simulink subsystem "ttc_on_road"  (R2022b)
settings: Solver=VariableStepAuto  StartTime=0.0  StopTime=10.0  RelTol=1e-3
settings Model: Creator=USER  LastModifiedBy=USER

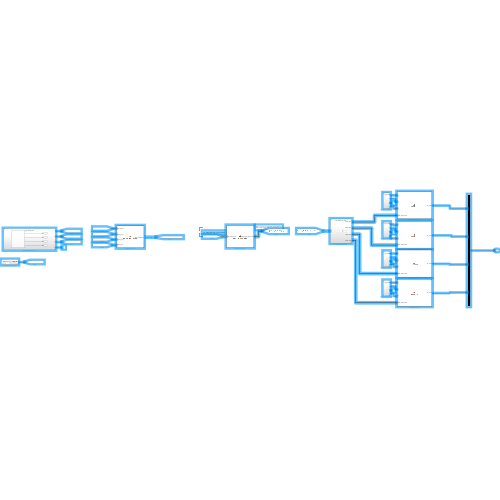
[thumbnail: Simulink's stored preview of the top-level diagram]
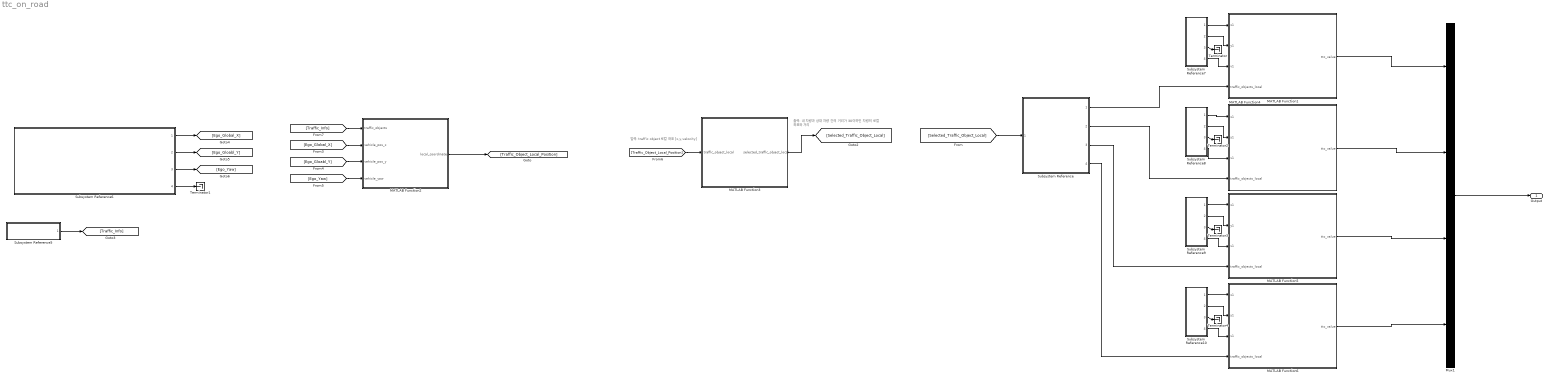
== system ttc_on_road ==
  note: 출력: 내 차량과 상대 차량 간의 거리가 30이하인 차령의 로컬 좌표와 거리
  note: 입력: traffic object 로컬 좌표 [x,y,velocity]
  MATLAB Function1 : MATLAB Function  TreatAsAtomicUnit=on
  MATLAB Function2 : MATLAB Function  TreatAsAtomicUnit=on
  MATLAB Function3 : MATLAB Function  TreatAsAtomicUnit=on
  MATLAB Function4 : MATLAB Function  TreatAsAtomicUnit=on
  MATLAB Function5 : MATLAB Function  TreatAsAtomicUnit=on
  MATLAB Function6 : MATLAB Function  TreatAsAtomicUnit=on
  Mux1 : Mux
  Subsystem Reference : Subsystem  ReferencedSubsystem=Get_Traffic_by_Line
  Subsystem Reference{6..10} (5 alike) : Subsystem  ReferencedSubsystem=ego_vehicle_info
  Subsystem Reference5 : Subsystem  ReferencedSubsystem=traffic_object_on_road_info
  Terminator{,1..4} (5 alike) : Terminator
  Output : Outport
  wires:
  Subsystem Reference7/4 -> MATLAB Function1/3(v1)
  Subsystem Reference7/1 -> MATLAB Function1/1(x1)
  MATLAB Function3/1(selected_traffic_object_local) -> [Selected_Traffic_Object_Local]
  MATLAB Function2/1(local_coordinates) -> [Traffic_Object_Local_Position]
  [Ego_Gloabl_Y] -> MATLAB Function2/3(vehicle_pos_y)
  Subsystem Reference6/3 -> [Ego_Yaw]
  [Traffic_Object_Local_Position] -> MATLAB Function3/1(traffic_object_local)
  Subsystem Reference10/1 -> MATLAB Function6/1(x1)
  MATLAB Function6/1(ttc_value) -> Mux1/4
  Subsystem Reference/1 -> MATLAB Function1/4(traffic_objects_local)
  Subsystem Reference/4 -> MATLAB Function6/4(traffic_objects_local)
  Subsystem Reference/2 -> MATLAB Function4/4(traffic_objects_local)
  Subsystem Reference8/2 -> MATLAB Function4/2(y1)
  Subsystem Reference7/3 -> Terminator/1
  Subsystem Reference8/4 -> MATLAB Function4/3(v1)
  Subsystem Reference9/3 -> Terminator3/1
  Subsystem Reference5/1 -> [Traffic_Info]
  Subsystem Reference10/3 -> Terminator4/1
  MATLAB Function4/1(ttc_value) -> Mux1/2
  Subsystem Reference8/1 -> MATLAB Function4/1(x1)
  MATLAB Function1/1(ttc_value) -> Mux1/1
  Subsystem Reference7/2 -> MATLAB Function1/2(y1)
  Subsystem Reference9/1 -> MATLAB Function5/1(x1)
  Subsystem Reference9/4 -> MATLAB Function5/3(v1)
  Subsystem Reference6/4 -> Terminator1/1
  Subsystem Reference/3 -> MATLAB Function5/4(traffic_objects_local)
  Mux1/1 -> Output/1
  Subsystem Reference6/2 -> [Ego_Gloabl_Y]
  Subsystem Reference9/2 -> MATLAB Function5/2(y1)
  [Ego_Yaw] -> MATLAB Function2/4(vehicle_yaw)
  Subsystem Reference8/3 -> Terminator2/1
  Subsystem Reference10/2 -> MATLAB Function6/2(y1)
  [Ego_Global_X] -> MATLAB Function2/2(vehicle_pos_x)
  MATLAB Function5/1(ttc_value) -> Mux1/3
  [Traffic_Info] -> MATLAB Function2/1(traffic_objects)
  Subsystem Reference6/1 -> [Ego_Global_X]
  Subsystem Reference10/4 -> MATLAB Function6/3(v1)
  [Selected_Traffic_Object_Local] -> Subsystem Reference/1

== matlab function ttc_on_road/MATLAB Function2 ==
  settings: updateMethod=DISCRETE  sampleTime=0.05
  data: local_coordinates output size=[30, 3]; traffic_objects input; vehicle_pos_x input; vehicle_pos_y input; vehicle_yaw input
function local_coordinates = global_to_local_position(traffic_objects, vehicle_pos_x, vehicle_pos_y, vehicle_yaw)
    % 차량 위치를 기준으로 변환 (평행 이동)
    delta_x = traffic_objects(:,1) - vehicle_pos_x;
    delta_y = traffic_objects(:,2) - vehicle_pos_y;
    
    % 차량의 요(방향)에 따른 회전 변환
    x_l = cos(vehicle_yaw) * delta_x + sin(vehicle_yaw) * delta_y;
    y_l = -sin(vehicle_yaw) * delta_x + cos(vehicle_yaw) * delta_y;
    
    coder.varsize('local_coordinates', [30, 3]);
    local_coordinates = zeros(size(traffic_objects,1),3); % 지역 좌표를 저장할 배열

    for i = 1:size(traffic_objects,1)
        velocity =  sqrt(traffic_objects(i,3)^2 + traffic_objects(i,4)^2);
        local_coordinates(i,:) = [x_l(i), y_l(i),velocity];
    end
end
% 
% function localVelocity = globalToLocalVelocity(v_x, v_y, theta)
%     % 전역 좌표계의 속도 벡터를 로컬 좌표계로 변환
%     %   v_x, v_y - 전역 좌표계에서의 속도 벡터 (x, y 속도)
%     %   theta - 차량의 진행 방향 (yaw angle in radians)
% 
%     v_x_l = cos(theta) * v_x + sin(theta) * v_y;
%     v_y_l = -sin(theta) * v_x + cos(theta) * v_y;
% 
%     % 회전 변환을 적용하여 로컬 속도를 계산
%     localVelocity =  sqrt(v_x_l^2 + v_y_l^2);
% end

== matlab function ttc_on_road/MATLAB Function3 ==
  settings: updateMethod=DISCRETE  sampleTime=0.05
  data: selected_traffic_object_local output size=[30, 4]; traffic_object_local input
function selected_traffic_object_local = select_near_traffic_object (traffic_object_local)
    % 차량 수
    numVehicles = size(traffic_object_local, 1);
    
    % 내 차와의 거리가 30 이하인 local cordinate를 저장할 배열
    coder.varsize('selected_traffic_object_local', [30, 4]);
    selected_traffic_object_local = zeros(0,4); 

    % 각 차량과의 거리 계산 및 거리가 30이하인 경우 출력으로 보냄
    for i = 1:numVehicles
        x = traffic_object_local(i,1);
        y = traffic_object_local(i,2);
        distance = sqrt(x^2 + y^2);

        if distance <= 30
            selected_traffic_object_local = [selected_traffic_object_local;traffic_object_local(i,:) distance];

        end
    end
end

== matlab function ttc_on_road/MATLAB Function4 ==
  settings: updateMethod=DISCRETE  sampleTime=0.05
  data: ttc_value output; x1 input; y1 input; v1 input; traffic_objects_local input
function ttc_value = calculateTTC(x1, y1, v1, traffic_objects_local)
    % 여러 상대 차량과의 Time to Collision 계산 함수
    % 입력:
    %   x1, y1 - 내 차량의 좌표
    %   v1 - 내 차량의 속도 (크기)
    %   traffic_objects_local - Nx3 행렬로, 각 행은 상대 차량의 (x, y,velocity) 좌표
    %   distance - Nx1 벡터로 내 차량과 다른 차량 사이의 거리
    % 출력:
    %   ttc_values - 각 상대 차량과의 Time to Collision 값

    % 차량 수
    numVehicles = size(traffic_objects_local, 1);

    if numVehicles > 0
        % 거리 및 TTC 저장을 위한 배열 초기화
        ttc_values = zeros(numVehicles, 1);
        
        % 각 차량과의 거리 및 상대 속도 계산
        for i = 1:numVehicles
    
            % 상대 속도 계산 (내 차량 속도와 상대 차량 속도의 차이)
            v2 = traffic_objects_local(i,3);
            relative_velocity = v2 - v1;

            % Time to Collision 계산
            if relative_velocity > 0
                ttc_values(i) = traffic_objects_local(i,4) / relative_velocity;
            else
                % 상대 속도가 0이거나 음수일 때 (멀어지는 경우 TTC는 무한대 처리)
                ttc_values(i) = inf;
            end
        end

        % 행렬에서 inf 값을 제외한 값들만 선택
        finiteValues = ttc_values(isfinite(ttc_values));
    
        % inf가 아닌 값들 중 최소 값 계산
        if ~isempty(finiteValues)
            ttc_value = min(finiteValues);
        else
            % 모든 값이 inf일 경우
            ttc_value = inf;
        end
    
    else
        ttc_value = inf;
    end
end

== matlab function ttc_on_road/MATLAB Function5 ==
  settings: updateMethod=DISCRETE  sampleTime=0.05
  data: ttc_value output; x1 input; y1 input; v1 input; traffic_objects_local input
function ttc_value = calculateTTC(x1, y1, v1, traffic_objects_local)
    % 여러 상대 차량과의 Time to Collision 계산 함수
    % 입력:
    %   x1, y1 - 내 차량의 좌표
    %   v1 - 내 차량의 속도 (크기)
    %   traffic_objects_local - Nx3 행렬로, 각 행은 상대 차량의 (x, y,velocity) 좌표
    %   distance - Nx1 벡터로 내 차량과 다른 차량 사이의 거리
    % 출력:
    %   ttc_values - 각 상대 차량과의 Time to Collision 값

    % 차량 수
    numVehicles = size(traffic_objects_local, 1);

    if numVehicles > 0
        % 거리 및 TTC 저장을 위한 배열 초기화
        ttc_values = zeros(numVehicles, 1);
        
        % 각 차량과의 거리 및 상대 속도 계산
        for i = 1:numVehicles
    
            % 상대 속도 계산 (내 차량 속도와 상대 차량 속도의 차이)
            v2 = traffic_objects_local(i,3);
            relative_velocity = v2 - v1;

            % Time to Collision 계산
            if relative_velocity > 0
                ttc_values(i) = traffic_objects_local(i,4) / relative_velocity;
            else
                % 상대 속도가 0이거나 음수일 때 (멀어지는 경우 TTC는 무한대 처리)
                ttc_values(i) = inf;
            end
        end

        % 행렬에서 inf 값을 제외한 값들만 선택
        finiteValues = ttc_values(isfinite(ttc_values));
    
        % inf가 아닌 값들 중 최소 값 계산
        if ~isempty(finiteValues)
            ttc_value = min(finiteValues);
        else
            % 모든 값이 inf일 경우
            ttc_value = inf;
        end
    
    else
        ttc_value = inf;
    end
end

== matlab function ttc_on_road/MATLAB Function6 ==
  settings: updateMethod=DISCRETE  sampleTime=0.05
  data: ttc_value output; x1 input; y1 input; v1 input; traffic_objects_local input
function ttc_value = calculateTTC(x1, y1, v1, traffic_objects_local)
    % 여러 상대 차량과의 Time to Collision 계산 함수
    % 입력:
    %   x1, y1 - 내 차량의 좌표
    %   v1 - 내 차량의 속도 (크기)
    %   traffic_objects_local - Nx3 행렬로, 각 행은 상대 차량의 (x, y,velocity) 좌표
    %   distance - Nx1 벡터로 내 차량과 다른 차량 사이의 거리
    % 출력:
    %   ttc_values - 각 상대 차량과의 Time to Collision 값

    % 차량 수
    numVehicles = size(traffic_objects_local, 1);

    if numVehicles > 0
        % 거리 및 TTC 저장을 위한 배열 초기화
        ttc_values = zeros(numVehicles, 1);
        
        % 각 차량과의 거리 및 상대 속도 계산
        for i = 1:numVehicles
    
            % 상대 속도 계산 (내 차량 속도와 상대 차량 속도의 차이)
            v2 = traffic_objects_local(i,3);
            relative_velocity = v2 - v1;

            % Time to Collision 계산
            if relative_velocity > 0
                ttc_values(i) = traffic_objects_local(i,4) / relative_velocity;
            else
                % 상대 속도가 0이거나 음수일 때 (멀어지는 경우 TTC는 무한대 처리)
                ttc_values(i) = inf;
            end
        end

        % 행렬에서 inf 값을 제외한 값들만 선택
        finiteValues = ttc_values(isfinite(ttc_values));
    
        % inf가 아닌 값들 중 최소 값 계산
        if ~isempty(finiteValues)
            ttc_value = min(finiteValues);
        else
            % 모든 값이 inf일 경우
            ttc_value = inf;
        end
    
    else
        ttc_value = inf;
    end
end

== matlab function ttc_on_road/MATLAB Function1 ==
  settings: updateMethod=DISCRETE  sampleTime=0.05
  data: ttc_value output; x1 input; y1 input; v1 input; traffic_objects_local input
function ttc_value = calculateTTC(x1, y1, v1, traffic_objects_local)
    % 여러 상대 차량과의 Time to Collision 계산 함수
    % 입력:
    %   x1, y1 - 내 차량의 좌표
    %   v1 - 내 차량의 속도 (크기)
    %   traffic_objects_local - Nx3 행렬로, 각 행은 상대 차량의 (x, y,velocity) 좌표
    %   distance - Nx1 벡터로 내 차량과 다른 차량 사이의 거리
    % 출력:
    %   ttc_values - 각 상대 차량과의 Time to Collision 값

    % 차량 수
    numVehicles = size(traffic_objects_local, 1);

    if numVehicles > 0
        % 거리 및 TTC 저장을 위한 배열 초기화
        ttc_values = zeros(numVehicles, 1);
        
        % 각 차량과의 거리 및 상대 속도 계산
        for i = 1:numVehicles
    
            % 상대 속도 계산 (내 차량 속도와 상대 차량 속도의 차이)
            v2 = traffic_objects_local(i,3);
            relative_velocity = v2 - v1;

            % Time to Collision 계산
            if relative_velocity > 0
                ttc_values(i) = traffic_objects_local(i,4) / relative_velocity;
            else
                % 상대 속도가 0이거나 음수일 때 (멀어지는 경우 TTC는 무한대 처리)
                ttc_values(i) = inf;
            end
        end

        % 행렬에서 inf 값을 제외한 값들만 선택
        finiteValues = ttc_values(isfinite(ttc_values));
    
        % inf가 아닌 값들 중 최소 값 계산
        if ~isempty(finiteValues)
            ttc_value = min(finiteValues);
        else
            % 모든 값이 inf일 경우
            ttc_value = inf;
        end
    
    else
        ttc_value = inf;
    end
end
